simulink library "servo_valve_pressure_control_module"  (R2025b)
settings: Solver=VariableStepAuto  StartTime=0.0  StopTime=10.0  RelTol=1e-3
libraries: slrealtimeloglib x1, SG_send_servo_valve_position_command x1
settings Model: Creator=cmmcguir  LastModifiedBy=cmmcguir

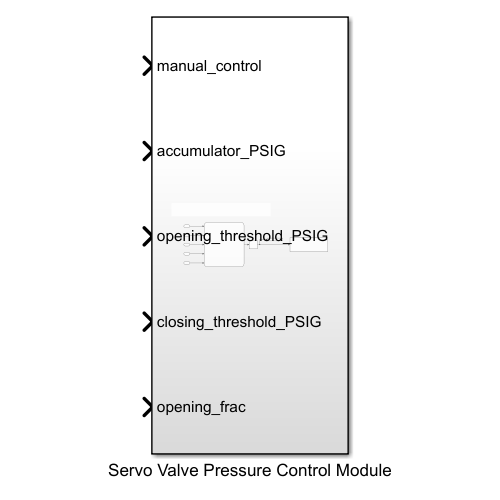
[thumbnail: Simulink's stored preview of the top-level diagram]
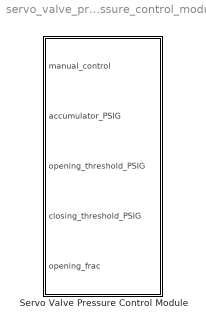
== system servo_valve_pressure_control_module ==
  Servo Valve Pressure Control Module : Subsystem

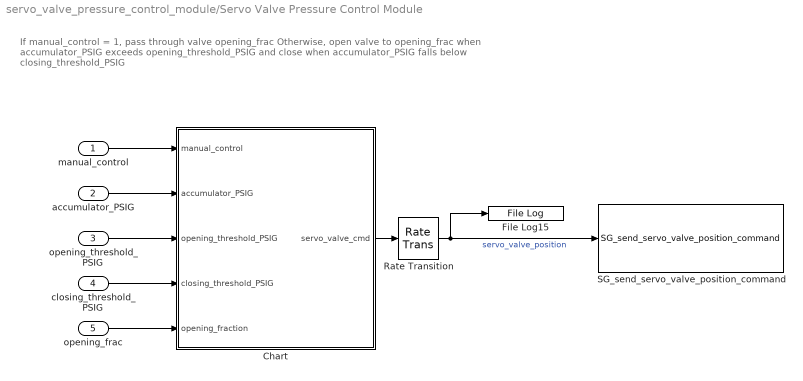
== system servo_valve_pressure_control_module/Servo Valve Pressure Control Module ==
  note: If manual_control = 1, pass through valve opening_frac
      |
      | Otherwise, open valve to opening_frac when accumulator_PSIG exceeds opening_threshold_PSIG
      | 	and close when accumulator_PSIG falls below closing_threshold_PSIG
  manual_control : Inport
  accumulator_PSIG : Inport  Port=2
  opening_threshold_PSIG : Inport  Port=3
  closing_threshold_PSIG : Inport  Port=4
  opening_frac : Inport  Port=5
  Chart : Stateflow chart  TreatAsAtomicUnit=on
  File Log15 : slrealtimeloglib/File Log  decimation=1  inputProcessing=Elements as channels (sample based)
  Rate Transition : RateTransition  OutPortSampleTime=0.01
  SG_send_servo_valve_position_command : SG_send_servo_valve_position_command/SG_send_servo_valve_position_command  SystemSampleTime=-1  VariantActivationTime=update diagram  EmptyChoice=off  PassThrough=off  PassThroughVariantControl=(default)  EmptyChoiceVariantControl=(default)  AllowFlexibleInterface=on  Latency=0  AutoFrameSizeCalculation=off
  wires:
  accumulator_PSIG/1 -> Chart/2(accumulator_PSIG)
  Chart/1(servo_valve_cmd) -> Rate Transition/1
  opening_frac/1 -> Chart/5(opening_fraction)
  Rate Transition/1 -> File Log15/1, SG_send_servo_valve_position_command/1  "servo_valve_position"
  closing_threshold_PSIG/1 -> Chart/4(closing_threshold_PSIG)
  opening_threshold_PSIG/1 -> Chart/3(opening_threshold_PSIG)
  manual_control/1 -> Chart/1(manual_control)

== stateflow chart servo_valve_pressure_control_module/Servo Valve Pressure Control Module/Chart ==
  state valve_init_1
    en:
    servo_valve_cmd = 0;
  state valve_init_2
    en:
    servo_valve_cmd = 0.1;
  state valve_closed
    en:
    servo_valve_cmd = 0;
  state manual_valve_control
    en, du:
    servo_valve_cmd = opening_fraction;
  state valve_opened
    en, du:
    servo_valve_cmd = opening_fraction;
  (default) -> valve_init_1
  valve_init_1 -> valve_init_2 : [after(0.1, sec)]
  valve_init_2 -> valve_closed : [after(0.1, sec)]
  manual_valve_control -> valve_closed : [~manual_control]
  valve_closed -> manual_valve_control [order 1] : [manual_control]
  (junction 19) -> manual_valve_control
  valve_closed -> valve_opened [order 2] : [accumulator_PSIG > opening_threshold_PSIG]
  valve_opened -> valve_closed [order 2] : [accumulator_PSIG < closing_threshold_PSIG]
  valve_opened -> (junction 19) [order 1] : [manual_control]
  data: manual_control input; accumulator_PSIG input size=1; opening_threshold_PSIG input size=1; closing_threshold_PSIG input size=1; opening_fraction input size=1; servo_valve_cmd output size=1
